simulink model "MassSpringDamper_model"  (R2025a)
settings: Solver=VariableStepAuto  StartTime=0.0  StopTime=50  RelTol=1e-3
values from neighbouring files (symbols this model uses):
  b = 1e-4    (= 0.0001)    [Static_Script.m]
  k = 28.10    (= 28.1)    [Static_Script.m]
  M = 0.336    [Static_Script.m]
undefined symbols (not defined in the file or in its folder): g
settings Model: Creator=User  LastModifiedBy=User

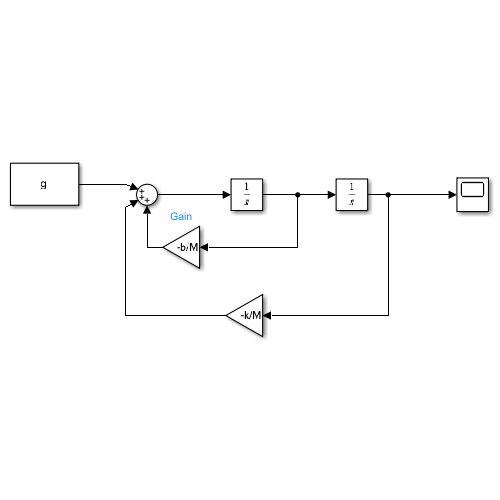
[thumbnail: Simulink's stored preview of the top-level diagram]
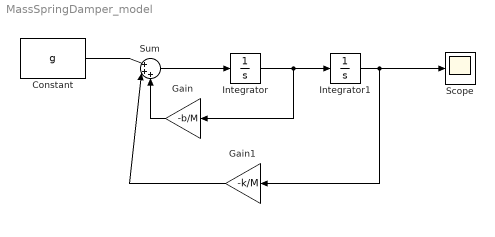
== system MassSpringDamper_model ==
  Constant : Constant  Value=g
  Gain : Gain  Gain=-b/M
  Gain1 : Gain  Gain=-k/M
  Integrator : Integrator
  Integrator1 : Integrator
  Scope : Scope
      settings: ActiveDisplayYMinimum=-9.1128866971552984  ActiveDisplayYMaximum=82.0159802743977
  Sum : Sum  Inputs=|+++
  wires:
  Constant/1 -> Sum/1
  Gain/1 -> Sum/3
  Gain1/1 -> Sum/2
  Sum/1 -> Integrator/1
  Integrator/1 -> Gain/1, Integrator1/1
  Integrator1/1 -> Gain1/1, Scope/1
